simulink model "PMDC_Panel_2018b"  (R2019b)
settings: Solver=ode45  StartTime=0.0  StopTime=0.2  RelTol=1e-6  AbsTol=1e-8
values from neighbouring files (symbols this model uses):
  b = 0.2    [PMDCMainprog.m]
  ba = alpha_s*J_hat - b_hat    (= 0.8)    [PMDCMainprog.m]
  H_c = 1/kp_c    (= 0.0357142857143)    [PMDCMainprog.m]
  H_s = 0    [PMDCMainprog.m]
  ia0 = 0    [PMDCMainprog.m]
  IconvLim = 23.7    [PMDCMainprog.m]
  J = 0.01    [PMDCMainprog.m]
  ki_c = alpha_c * (Ra + R_hat)    (= 28000)    [PMDCMainprog.m]
  ki_s = alpha_s * (ba + b_hat)    (= 100)    [PMDCMainprog.m]
  kp_c = alpha_c * L_hat    (= 28)    [PMDCMainprog.m]
  kp_s = alpha_s  * J_hat    (= 1)    [PMDCMainprog.m]
  L = 0.028    [PMDCMainprog.m]
  nstep = 1000    [PMDCMainprog.m]
  nstep_time = 0.001    [PMDCMainprog.m]
  Psy = 1.242    [PMDCMainprog.m]
  R = 1.68    [PMDCMainprog.m]
  Ra = alpha_c*L_hat - R_hat    (= 26.32)    [PMDCMainprog.m]
  rpm_to_rad_s = 2*pi/60    (= 0.10471975512)    [PMDCMainprog.m]
  tstep = 10    [PMDCMainprog.m]
  tstep_time_1 = 0.2    [PMDCMainprog.m]
  tstep_time_2 = 0.3    [PMDCMainprog.m]
  VconvLim = inf    [PMDCMainprog.m]
settings Model: ExtModeTrigMode=oneshot  ExtModeArmWhenConnect=off  ExtModeAutoUpdateStatusClock=off  Creator=e6zebra  LastModifiedBy=smitd
settings SolverCC: AutoScaleAbsTol=off
settings DataIOCC: SaveFormat=Array  SignalLoggingSaveFormat=ModelDataLogs  ReturnWorkspaceOutputs=off
settings OptimizationCC: BlockReduction=off  BooleanDataType=off  ExpressionDepthLimit=2147483647  InitFltsAndDblsToZero=on  LifeSpan=inf
settings DebuggingCC: SaveWithParameterizedLinksMsg=none  UnderspecifiedInitializationDetection=Classic  MergeDetectMultiDrivingBlocksExec=none  SignalResolutionControl=TryResolveAllWithWarning  MultiTaskDSMMsg=warning  MultiTaskCondExecSysMsg=none  FcnCallInpInsideContextMsg=warning  StateNameClashWarn=warning  SFUnexpectedBacktrackingDiag=warning  SFNoUnconditionalDefaultTransitionDiag=warning  SFExecutionAtInitializationDiag=none  ArithmeticOperatorsInVariantConditions=warning
settings HardwareCC: ProdBitPerPointer=32  ProdBitPerSizeT=32  ProdBitPerPtrDiffT=32  ProdLargestAtomicFloat=None  ProdIntDivRoundTo=Undefined  ProdEndianess=Unspecified  ProdWordSize=32  ProdHWDeviceType=32-bit Generic  TargetUnknown=on
settings ModelReferenceCC: PropagateSignalLabelsOutOfModel=off
settings SFSimCC: SimUseLocalCustomCode=off  CustomCodeUndefinedFunction=UseInterfaceOnly
settings RTWCC: TemplateMakefile=grt.tmf  RTWUseLocalCustomCode=off
settings CodeAppCC: StateflowObjectComments=on
settings GRTTargetCC: TargetFcnLib=ansi_tfl_tmw.mat  TargetLangStandard=C89/C90 (ANSI)  GeneratePreprocessorConditionals=Disable all  CombineOutputUpdateFcns=off  GRTInterface=on
settings ConfigComp: CovMetricSettings=dw  CovHtmlReporting=on  CovSaveCumulativeToWorkspaceVar=on  CovSaveSingleToWorkspaceVar=on  CovExternalEMLEnable=off  CovSFcnEnable=off

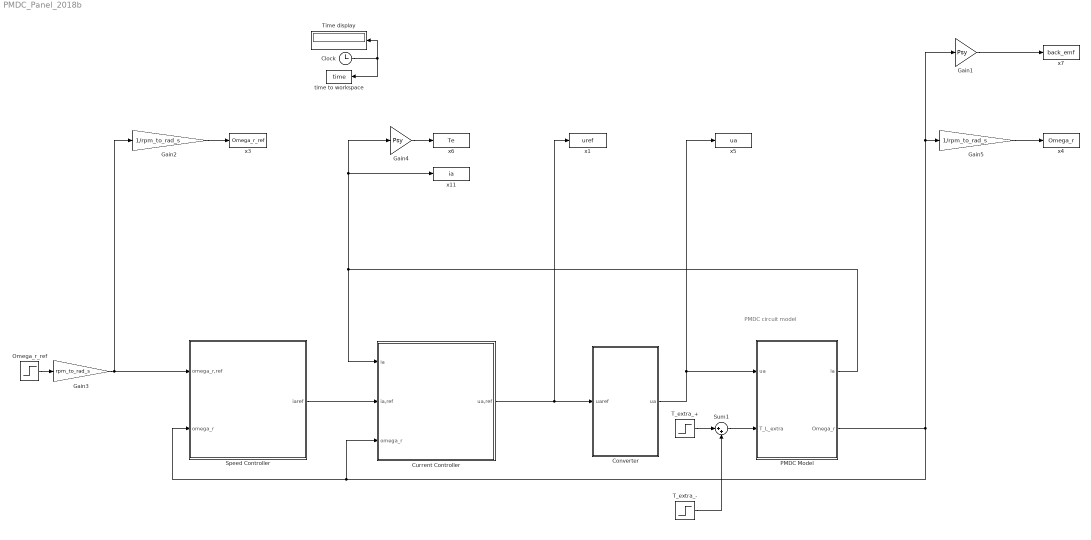
== system PMDC_Panel_2018b ==
  note: PMDC circuit model
  Clock : Clock
  Converter : Subsystem
  Current Controller : Subsystem
  Gain1 : Gain  Gain=Psy
  Gain2 : Gain  Gain=1/rpm_to_rad_s
  Gain3 : Gain  Gain=rpm_to_rad_s
  Gain4 : Gain  Gain=Psy
  Gain5 : Gain  Gain=1/rpm_to_rad_s
  "Omega_r_ref " : Step  Time=nstep_time  After=nstep  SampleTime=0
  PMDC Model : Subsystem
  Speed Controller : Subsystem
  Sum1 : Sum  Inputs=|++
  T_extra_+ : Step  Time=tstep_time_1  After=tstep  SampleTime=0
  T_extra_- : Step  Time=tstep_time_2  After=-tstep  SampleTime=0
  Time display : Display
  time to workspace : ToWorkspace  VariableName=time  SampleTime=-1
  x1 : ToWorkspace  VariableName=uref  SampleTime=-1
  x11 : ToWorkspace  VariableName=ia  SampleTime=-1
  x3 : ToWorkspace  VariableName=Omega_r_ref  SampleTime=-1
  x4 : ToWorkspace  VariableName=Omega_r  SampleTime=-1
  x5 : ToWorkspace  VariableName=ua  SampleTime=-1
  x6 : ToWorkspace  VariableName=Te  SampleTime=-1
  x7 : ToWorkspace  VariableName=back_emf  SampleTime=-1
  wires:
  Clock/1 -> Time display/1, time to workspace/1
  Converter/1(ua) -> x5/1, PMDC Model/1(ua)
  Speed Controller/1(iaref) -> Current Controller/2(ia,ref)
  "Omega_r_ref "/1 -> Gain3/1
  Gain4/1 -> x6/1
  Gain1/1 -> x7/1
  Current Controller/1(ua,ref) -> x1/1, Converter/1(uaref)
  Sum1/1 -> PMDC Model/2(T_L_extra)
  T_extra_+/1 -> Sum1/1
  T_extra_-/1 -> Sum1/2
  PMDC Model/2(Omega_r) -> Gain5/1, Gain1/1, Current Controller/3(omega_r), Speed Controller/2(omega_r)
  Gain3/1 -> Gain2/1, Speed Controller/1(omega_r,ref)
  Gain2/1 -> x3/1
  Gain5/1 -> x4/1
  PMDC Model/1(ia) -> Current Controller/1(ia), x11/1, Gain4/1

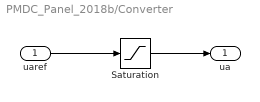
== system PMDC_Panel_2018b/Converter ==
  uaref : Inport
  Saturation : Saturate  UpperLimit=VconvLim  LowerLimit=-VconvLim
  ua : Outport  VectorParamsAs1DForOutWhenUnconnected=off
  wires:
  Saturation/1 -> ua/1
  uaref/1 -> Saturation/1

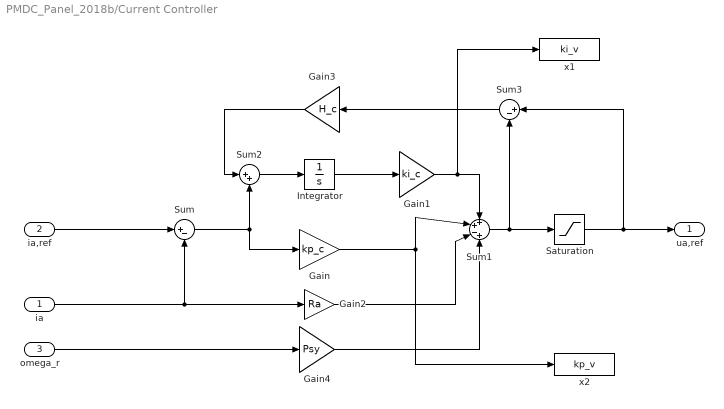
== system PMDC_Panel_2018b/Current Controller ==
  ia : Inport
  ia,ref : Inport  Port=2
  omega_r : Inport  Port=3
  Gain : Gain  Gain=kp_c
  Gain1 : Gain  Gain=ki_c
  Gain2 : Gain  Gain=Ra
  Gain3 : Gain  Gain=H_c
  Gain4 : Gain  Gain=Psy
  Integrator : Integrator
  Saturation : Saturate  UpperLimit=VconvLim  LowerLimit=-VconvLim
  Sum : Sum  Inputs=|+-
  Sum1 : Sum  Inputs=++-+
  Sum2 : Sum  Inputs=|++
  Sum3 : Sum  Inputs=|+-
  x1 : ToWorkspace  VariableName=ki_v  SampleTime=-1
  x2 : ToWorkspace  VariableName=kp_v  SampleTime=-1
  ua,ref : Outport  VectorParamsAs1DForOutWhenUnconnected=off
  wires:
  ia/1 -> Gain2/1, Sum/2
  Sum/1 -> Sum2/2, Gain/1
  Integrator/1 -> Gain1/1
  Gain2/1 -> Sum1/3
  Sum2/1 -> Integrator/1
  Gain3/1 -> Sum2/1
  Gain/1 -> Sum1/2, x2/1
  Gain1/1 -> x1/1, Sum1/1
  Sum1/1 -> Saturation/1, Sum3/2
  Saturation/1 -> Sum3/1, ua,ref/1
  Sum3/1 -> Gain3/1
  ia,ref/1 -> Sum/1
  omega_r/1 -> Gain4/1
  Gain4/1 -> Sum1/4

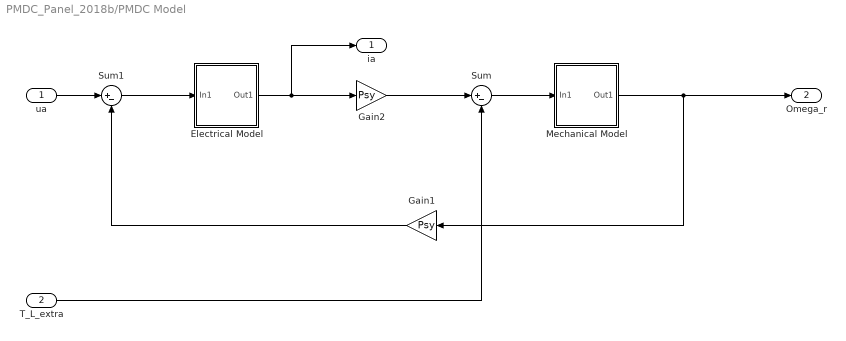
== system PMDC_Panel_2018b/PMDC Model ==
  ua : Inport
  T_L_extra : Inport  Port=2
  Electrical Model : Subsystem
  Gain1 : Gain  Gain=Psy
  Gain2 : Gain  Gain=Psy
  Mechanical Model : Subsystem
  Sum : Sum  Inputs=|+-
  Sum1 : Sum  Inputs=|+-
  ia : Outport  VectorParamsAs1DForOutWhenUnconnected=off
  Omega_r : Outport  Port=2  VectorParamsAs1DForOutWhenUnconnected=off
  wires:
  Electrical Model/1(Out1) -> Gain2/1, ia/1
  Gain2/1 -> Sum/1
  T_L_extra/1 -> Sum/2
  Sum/1 -> Mechanical Model/1(In1)
  Mechanical Model/1(Out1) -> Gain1/1, Omega_r/1
  ua/1 -> Sum1/1
  Sum1/1 -> Electrical Model/1(In1)
  Gain1/1 -> Sum1/2

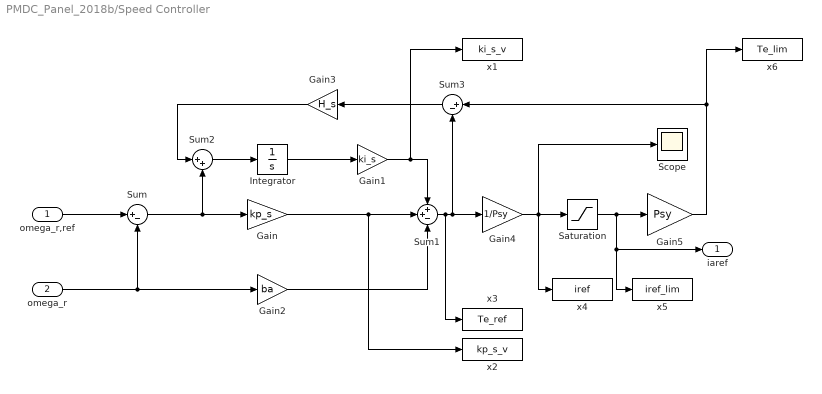
== system PMDC_Panel_2018b/Speed Controller ==
  omega_r,ref : Inport
  omega_r : Inport  Port=2
  Gain : Gain  Gain=kp_s
  Gain1 : Gain  Gain=ki_s
  Gain2 : Gain  Gain=ba
  Gain3 : Gain  Gain=H_s
  Gain4 : Gain  Gain=1/Psy
  Gain5 : Gain  Gain=Psy
  Integrator : Integrator
  Saturation : Saturate  UpperLimit=IconvLim  LowerLimit=-IconvLim
  Scope : Scope
  Sum : Sum  Inputs=|+-
  Sum1 : Sum  Inputs=++-
  Sum2 : Sum  Inputs=|++
  Sum3 : Sum  Inputs=|+-
  x1 : ToWorkspace  VariableName=ki_s_v  SampleTime=-1
  x2 : ToWorkspace  VariableName=kp_s_v  SampleTime=-1
  x3 : ToWorkspace  VariableName=Te_ref  SampleTime=-1
  x4 : ToWorkspace  VariableName=iref  SampleTime=-1
  x5 : ToWorkspace  VariableName=iref_lim  SampleTime=-1
  x6 : ToWorkspace  VariableName=Te_lim  SampleTime=-1
  iaref : Outport  VectorParamsAs1DForOutWhenUnconnected=off
  wires:
  Sum3/1 -> Gain3/1
  Gain1/1 -> Sum1/1, x1/1
  Gain/1 -> Sum1/2, x2/1
  Gain3/1 -> Sum2/1
  Sum2/1 -> Integrator/1
  Gain2/1 -> Sum1/3
  Integrator/1 -> Gain1/1
  Sum/1 -> Gain/1, Sum2/2
  omega_r/1 -> Sum/2, Gain2/1
  omega_r,ref/1 -> Sum/1
  Saturation/1 -> iaref/1, x5/1, Gain5/1
  Gain4/1 -> x4/1, Scope/1, Saturation/1
  Sum1/1 -> x3/1, Gain4/1, Sum3/2
  Gain5/1 -> Sum3/1, x6/1

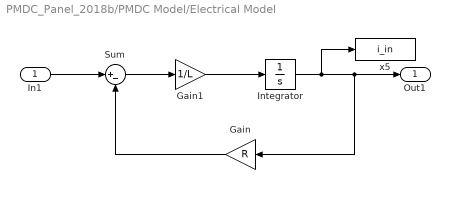
== system PMDC_Panel_2018b/PMDC Model/Electrical Model ==
  In1 : Inport
  Gain : Gain  Gain=R
  Gain1 : Gain  Gain=1/L
  Integrator : Integrator  InitialCondition=ia0
  Sum : Sum  Inputs=|+-
  x5 : ToWorkspace  VariableName=i_in  SampleTime=-1
  Out1 : Outport
  wires:
  Integrator/1 -> x5/1, Out1/1, Gain/1
  Sum/1 -> Gain1/1
  Gain/1 -> Sum/2
  In1/1 -> Sum/1
  Gain1/1 -> Integrator/1

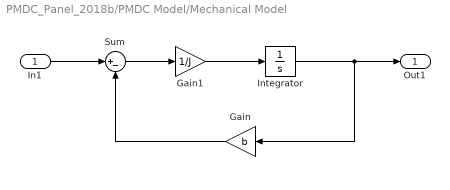
== system PMDC_Panel_2018b/PMDC Model/Mechanical Model ==
  In1 : Inport
  Gain : Gain  Gain=b
  Gain1 : Gain  Gain=1/J
  Integrator : Integrator  InitialCondition=ia0
  Sum : Sum  Inputs=|+-
  Out1 : Outport
  wires:
  Integrator/1 -> Out1/1, Gain/1
  Sum/1 -> Gain1/1
  Gain/1 -> Sum/2
  In1/1 -> Sum/1
  Gain1/1 -> Integrator/1
